simulink model "comparisonModel"  (R2017b)
settings: Solver=VariableStepAuto  StartTime=0.0  StopTime=100  RelTol=1e-3
undefined symbols (not defined in the file): DiscIntNeverNeededParam, sigbuilder_block
settings Model: Creator=Matthias  LastModifiedBy=Kris
settings DebuggingCC: ModelReferenceExtraNoncontSigs=none

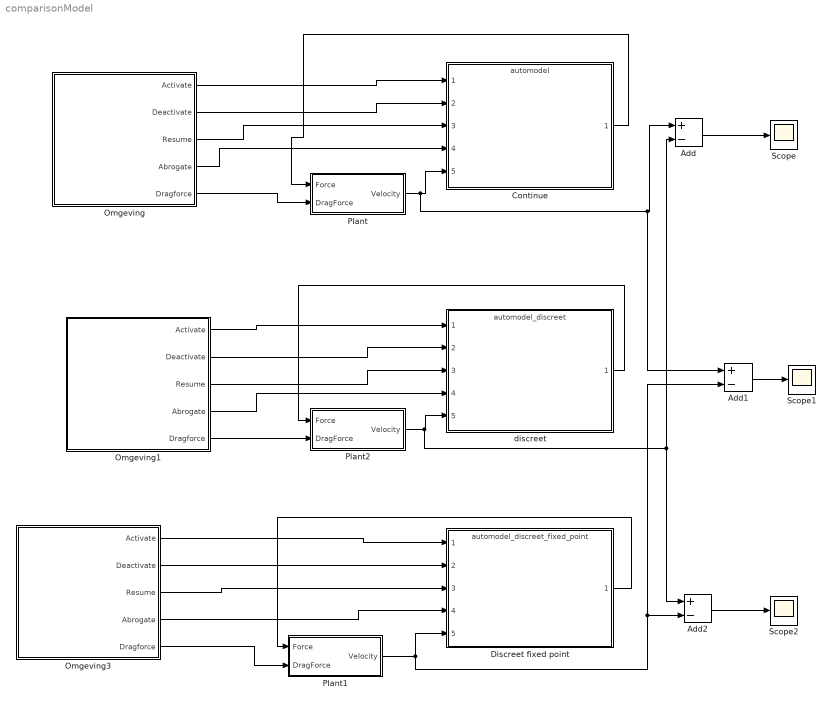
== system comparisonModel ==
  Add : Sum  Inputs=+-
  Add1 : Sum  Inputs=+-
  Add2 : Sum  Inputs=+-
  Continue : ModelReference  ModelNameDialog=automodel.slx  SimulationMode=Normal  ModelReferenceVersion=1.46
  Discreet fixed point : ModelReference  ModelNameDialog=automodel_discreet_fixed_point.slx  SimulationMode=Normal  ModelReferenceVersion=1.55
  Omgeving : Subsystem
  Omgeving1 : Subsystem
  Omgeving3 : Subsystem
  Plant : Subsystem
  Plant1 : Subsystem
  Plant2 : Subsystem
  Scope : Scope
  Scope1 : Scope
  Scope2 : Scope
  discreet : ModelReference  ModelNameDialog=automodel_discreet.slx  SimulationMode=Normal  ModelReferenceVersion=1.47
  wires:
  Omgeving/4(Abrogate) -> Continue/4
  Omgeving/3(Resume) -> Continue/3
  Omgeving/2(Deactivate) -> Continue/2
  Omgeving/1(Activate) -> Continue/1
  Add/1 -> Scope/1
  Add1/1 -> Scope1/1
  Add2/1 -> Scope2/1
  Plant/1(Velocity) -> Add1/1, Add/1, Continue/5
  Plant2/1(Velocity) -> Add/2, Add2/1, discreet/5
  Omgeving1/1(Activate) -> discreet/1
  Omgeving1/2(Deactivate) -> discreet/2
  Omgeving1/3(Resume) -> discreet/3
  Omgeving1/4(Abrogate) -> discreet/4
  Omgeving1/5(Dragforce) -> Plant2/2(DragForce)
  Omgeving/5(Dragforce) -> Plant/2(DragForce)
  Omgeving3/5(Dragforce) -> Plant1/2(DragForce)
  Omgeving3/1(Activate) -> Discreet fixed point/1
  Discreet fixed point/1 -> Plant1/1("Force ")
  Omgeving3/2(Deactivate) -> Discreet fixed point/2
  Omgeving3/4(Abrogate) -> Discreet fixed point/4
  Omgeving3/3(Resume) -> Discreet fixed point/3
  Plant1/1(Velocity) -> Add2/2, Add1/2, Discreet fixed point/5
  discreet/1 -> Plant2/1("Force ")
  Continue/1 -> Plant/1("Force ")

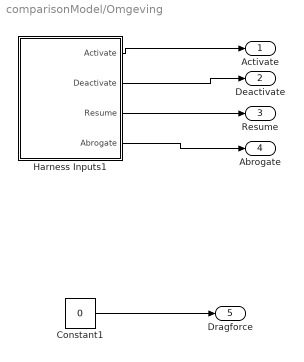
== system comparisonModel/Omgeving ==
  Constant1 : Constant  Value=0
  Harness Inputs1 : Subsystem  Tag=STV Subsys  LoadFcn=sigbuilder_block('load');  StartFcn=sigbuilder_block('start');  StopFcn=sigbuilder_block('stop');  ClipboardFcn=sigbuilder_block('clipboard');  mask(Sigbuilder block){tuvar=[0:10]}
      mask init:
      | if ~strcmp(get_param(bdroot(gcb),'SimulationStatus'),'stopped'),tuvar = sigbuilder_block('maskInit'); end
      settings: CopyFcn=sigbuilder_block('copy');  DeleteFcn=sigbuilder_block('delete');  ModelCloseFcn=sigbuilder_block('modelClose');  PreSaveFcn=sigbuilder_block('preSave');  PauseFcn=sigbuilder_block('pause');  ContinueFcn=sigbuilder_block('continue');  NameChangeFcn=sigbuilder_block('namechange');  OpenFcn=sigbuilder_block('open',[50.25 50.25 878.25 399.75 ]);  CloseFcn=sigbuilder_block('close');
      mask Display: plot(0, 0, 100, 100,[2, 2, 32, 32, 2], [68, 8, 8, 68, 68],[32, 2], [38, 38], [32, 19, 2],[53, 60, 44], [32, 17, 17, 2],[16, 16, 31, 31]);txt = getActiveGroup(gcbh);text(2, 100, txt,'verticalAlignment', 'top');
  Activate : Outport
  Deactivate : Outport  Port=2
  Resume : Outport  Port=3
  Abrogate : Outport  Port=4
  Dragforce : Outport  Port=5
  wires:
  Harness Inputs1/1(Activate) -> Activate/1
  Harness Inputs1/2(Deactivate) -> Deactivate/1
  Harness Inputs1/3(Resume) -> Resume/1
  Harness Inputs1/4(Abrogate) -> Abrogate/1
  Constant1/1 -> Dragforce/1

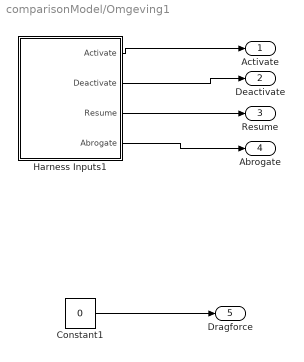
== system comparisonModel/Omgeving1 ==
  Constant1 : Constant  Value=0
  Harness Inputs1 : Subsystem  Tag=STV Subsys  LoadFcn=sigbuilder_block('load');  StartFcn=sigbuilder_block('start');  StopFcn=sigbuilder_block('stop');  ClipboardFcn=sigbuilder_block('clipboard');  mask(Sigbuilder block){tuvar=[0:10]}
      mask init:
      | if ~strcmp(get_param(bdroot(gcb),'SimulationStatus'),'stopped'),tuvar = sigbuilder_block('maskInit'); end
      settings: CopyFcn=sigbuilder_block('copy');  DeleteFcn=sigbuilder_block('delete');  ModelCloseFcn=sigbuilder_block('modelClose');  PreSaveFcn=sigbuilder_block('preSave');  PauseFcn=sigbuilder_block('pause');  ContinueFcn=sigbuilder_block('continue');  NameChangeFcn=sigbuilder_block('namechange');  OpenFcn=sigbuilder_block('open',[50.25 50.25 878.25 399.75 ]);  CloseFcn=sigbuilder_block('close');
      mask Display: plot(0, 0, 100, 100,[2, 2, 32, 32, 2], [68, 8, 8, 68, 68],[32, 2], [38, 38], [32, 19, 2],[53, 60, 44], [32, 17, 17, 2],[16, 16, 31, 31]);txt = getActiveGroup(gcbh);text(2, 100, txt,'verticalAlignment', 'top');
  Activate : Outport
  Deactivate : Outport  Port=2
  Resume : Outport  Port=3
  Abrogate : Outport  Port=4
  Dragforce : Outport  Port=5
  wires:
  Harness Inputs1/1(Activate) -> Activate/1
  Harness Inputs1/2(Deactivate) -> Deactivate/1
  Harness Inputs1/3(Resume) -> Resume/1
  Harness Inputs1/4(Abrogate) -> Abrogate/1
  Constant1/1 -> Dragforce/1

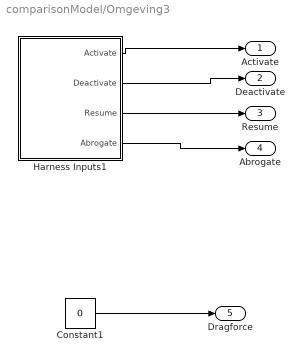
== system comparisonModel/Omgeving3 ==
  Constant1 : Constant  Value=0
  Harness Inputs1 : Subsystem  Tag=STV Subsys  LoadFcn=sigbuilder_block('load');  StartFcn=sigbuilder_block('start');  StopFcn=sigbuilder_block('stop');  ClipboardFcn=sigbuilder_block('clipboard');  mask(Sigbuilder block){tuvar=[0:10]}
      mask init:
      | if ~strcmp(get_param(bdroot(gcb),'SimulationStatus'),'stopped'),tuvar = sigbuilder_block('maskInit'); end
      settings: CopyFcn=sigbuilder_block('copy');  DeleteFcn=sigbuilder_block('delete');  ModelCloseFcn=sigbuilder_block('modelClose');  PreSaveFcn=sigbuilder_block('preSave');  PauseFcn=sigbuilder_block('pause');  ContinueFcn=sigbuilder_block('continue');  NameChangeFcn=sigbuilder_block('namechange');  OpenFcn=sigbuilder_block('open',[50.25 50.25 878.25 399.75 ]);  CloseFcn=sigbuilder_block('close');
      mask Display: plot(0, 0, 100, 100,[2, 2, 32, 32, 2], [68, 8, 8, 68, 68],[32, 2], [38, 38], [32, 19, 2],[53, 60, 44], [32, 17, 17, 2],[16, 16, 31, 31]);txt = getActiveGroup(gcbh);text(2, 100, txt,'verticalAlignment', 'top');
  Activate : Outport
  Deactivate : Outport  Port=2
  Resume : Outport  Port=3
  Abrogate : Outport  Port=4
  Dragforce : Outport  Port=5
  wires:
  Harness Inputs1/1(Activate) -> Activate/1
  Harness Inputs1/2(Deactivate) -> Deactivate/1
  Harness Inputs1/3(Resume) -> Resume/1
  Harness Inputs1/4(Abrogate) -> Abrogate/1
  Constant1/1 -> Dragforce/1

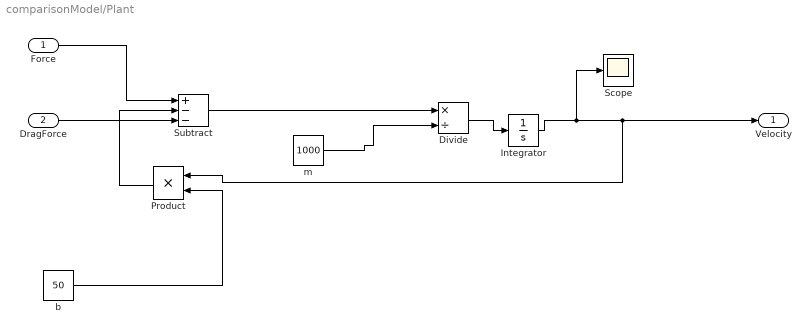
== system comparisonModel/Plant ==
  "Force " : Inport
  DragForce : Inport  Port=2
  Divide : Product  Inputs=*/
  Integrator : Integrator
  Product : Product
  Scope : Scope
  Subtract : Sum  Inputs=+--
  b : Constant  Value=50
  m : Constant  Value=1000
  Velocity : Outport
  wires:
  Product/1 -> Subtract/2
  b/1 -> Product/2
  Subtract/1 -> Divide/1
  "Force "/1 -> Subtract/1
  Divide/1 -> Integrator/1
  m/1 -> Divide/2
  DragForce/1 -> Subtract/3
  Integrator/1 -> Scope/1, Product/1, Velocity/1

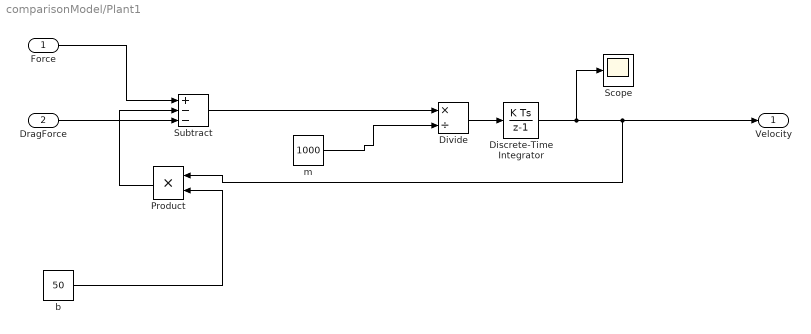
== system comparisonModel/Plant1 ==
  "Force " : Inport
  DragForce : Inport  Port=2
  Discrete-Time Integrator : DiscreteIntegrator  InitialConditionSetting=State (most efficient)  SampleTime=-1  OutDataTypeStr=Inherit: Inherit via back propagation  ICPrevOutput=DiscIntNeverNeededParam  ICPrevScaledInput=DiscIntNeverNeededParam
  Divide : Product  Inputs=*/  OutDataTypeStr=Inherit: Inherit via back propagation
  Product : Product
  Scope : Scope
  Subtract : Sum  Inputs=+--
  b : Constant  Value=50  OutDataTypeStr=fixdt(1,32,0)
  m : Constant  Value=1000
  Velocity : Outport
  wires:
  Product/1 -> Subtract/2
  b/1 -> Product/2
  Subtract/1 -> Divide/1
  "Force "/1 -> Subtract/1
  Divide/1 -> Discrete-Time Integrator/1
  m/1 -> Divide/2
  DragForce/1 -> Subtract/3
  Discrete-Time Integrator/1 -> Scope/1, Product/1, Velocity/1

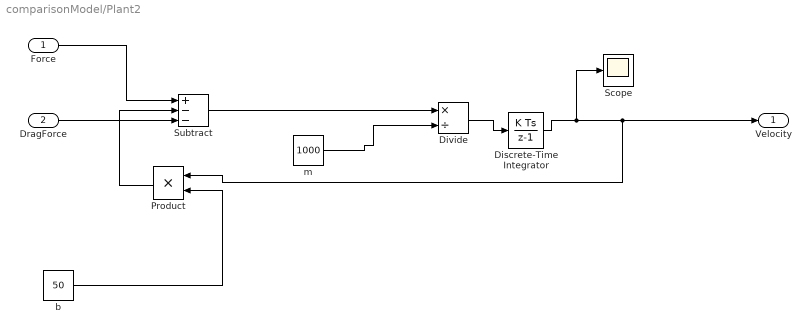
== system comparisonModel/Plant2 ==
  "Force " : Inport
  DragForce : Inport  Port=2
  Discrete-Time Integrator : DiscreteIntegrator  InitialConditionSetting=State (most efficient)  SampleTime=-1  ICPrevOutput=DiscIntNeverNeededParam  ICPrevScaledInput=DiscIntNeverNeededParam
  Divide : Product  Inputs=*/
  Product : Product
  Scope : Scope
  Subtract : Sum  Inputs=+--
  b : Constant  Value=50
  m : Constant  Value=1000
  Velocity : Outport
  wires:
  Product/1 -> Subtract/2
  b/1 -> Product/2
  Subtract/1 -> Divide/1
  "Force "/1 -> Subtract/1
  Divide/1 -> Discrete-Time Integrator/1
  m/1 -> Divide/2
  DragForce/1 -> Subtract/3
  Discrete-Time Integrator/1 -> Scope/1, Product/1, Velocity/1

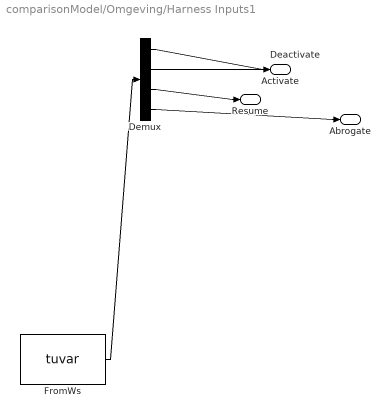
== system comparisonModel/Omgeving/Harness Inputs1 ==
  Demux : Demux  Tag=STV Demux
  FromWs : FromWorkspace  Tag=STV FromWs  VariableName=tuvar  SampleTime=0
      SigBuilderData=|
      | dataSet.timeRange = [0 200]
      | dataSet.name = 'Group 1'
      | sbobj.Name = 'Signal Builder'
      | sbobj.Groups.Name = 'Group 1'
      | sbobj.Groups.Signals(1).Name = 'Activate'
      | sbobj.Groups.Signals(1).XData = [0 7.2 7.2 200]
      | sbobj.Groups.Signals(1).YData = [0 0 1 1]
      | sbobj.Groups.Signals(2).Name = 'Deactivate'
      | sbobj.Groups.Signals(2).XData = [0 0.1 200]
      | sbobj.Groups.Signals(2).YData = [0 0 0]
      | sbobj.Groups.Signals(3).Name = 'Resume'
      | sbobj.Groups.Signals(3).XData = [0 200]
      | sbobj.Groups.Signals(3).YData = [0 0]
      | sbobj.Groups.Signals(4).Name = 'Abrogate'
      | sbobj.Groups.Signals(4).XData = [0 200]
      | sbobj.Groups.Signals(4).YData = [0 0]
      | sbobj.Groups.TimeRange = [0 200]
  Activate : Outport  Tag=STV Outport
  Deactivate : Outport  Tag=STV Outport  Port=2
  Resume : Outport  Tag=STV Outport  Port=3
  Abrogate : Outport  Tag=STV Outport  Port=4
  wires:
  FromWs/1 -> Demux/1
  Demux/1 -> Activate/1
  Demux/2 -> Deactivate/1
  Demux/3 -> Resume/1
  Demux/4 -> Abrogate/1

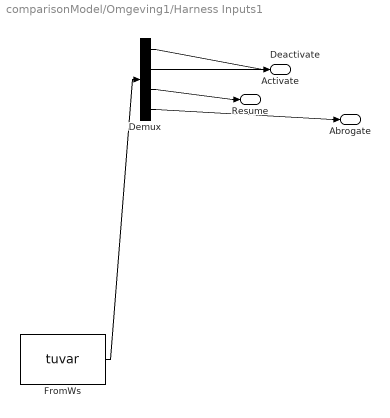
== system comparisonModel/Omgeving1/Harness Inputs1 ==
  Demux : Demux  Tag=STV Demux
  FromWs : FromWorkspace  Tag=STV FromWs  VariableName=tuvar  SampleTime=0
      SigBuilderData=|
      | dataSet.timeRange = [0 200]
      | dataSet.name = 'Group 1'
      | sbobj.Name = 'Signal Builder'
      | sbobj.Groups.Name = 'Group 1'
      | sbobj.Groups.Signals(1).Name = 'Activate'
      | sbobj.Groups.Signals(1).XData = [0 7.2 7.2 200]
      | sbobj.Groups.Signals(1).YData = [0 0 1 1]
      | sbobj.Groups.Signals(2).Name = 'Deactivate'
      | sbobj.Groups.Signals(2).XData = [0 0.1 200]
      | sbobj.Groups.Signals(2).YData = [0 0 0]
      | sbobj.Groups.Signals(3).Name = 'Resume'
      | sbobj.Groups.Signals(3).XData = [0 200]
      | sbobj.Groups.Signals(3).YData = [0 0]
      | sbobj.Groups.Signals(4).Name = 'Abrogate'
      | sbobj.Groups.Signals(4).XData = [0 200]
      | sbobj.Groups.Signals(4).YData = [0 0]
      | sbobj.Groups.TimeRange = [0 200]
  Activate : Outport  Tag=STV Outport
  Deactivate : Outport  Tag=STV Outport  Port=2
  Resume : Outport  Tag=STV Outport  Port=3
  Abrogate : Outport  Tag=STV Outport  Port=4
  wires:
  FromWs/1 -> Demux/1
  Demux/1 -> Activate/1
  Demux/2 -> Deactivate/1
  Demux/3 -> Resume/1
  Demux/4 -> Abrogate/1

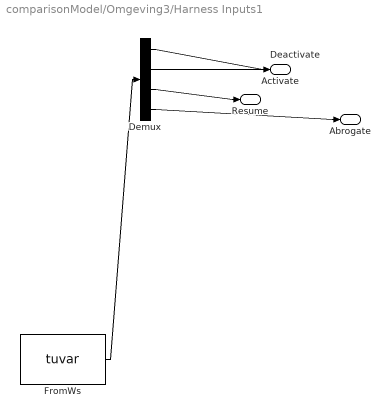
== system comparisonModel/Omgeving3/Harness Inputs1 ==
  Demux : Demux  Tag=STV Demux
  FromWs : FromWorkspace  Tag=STV FromWs  VariableName=tuvar  SampleTime=0
      SigBuilderData=|
      | dataSet.timeRange = [0 200]
      | dataSet.name = 'Group 1'
      | sbobj.Name = 'Signal Builder'
      | sbobj.Groups.Name = 'Group 1'
      | sbobj.Groups.Signals(1).Name = 'Activate'
      | sbobj.Groups.Signals(1).XData = [0 7.2 7.2 200]
      | sbobj.Groups.Signals(1).YData = [0 0 1 1]
      | sbobj.Groups.Signals(2).Name = 'Deactivate'
      | sbobj.Groups.Signals(2).XData = [0 0.1 200]
      | sbobj.Groups.Signals(2).YData = [0 0 0]
      | sbobj.Groups.Signals(3).Name = 'Resume'
      | sbobj.Groups.Signals(3).XData = [0 200]
      | sbobj.Groups.Signals(3).YData = [0 0]
      | sbobj.Groups.Signals(4).Name = 'Abrogate'
      | sbobj.Groups.Signals(4).XData = [0 200]
      | sbobj.Groups.Signals(4).YData = [0 0]
      | sbobj.Groups.TimeRange = [0 200]
  Activate : Outport  Tag=STV Outport
  Deactivate : Outport  Tag=STV Outport  Port=2
  Resume : Outport  Tag=STV Outport  Port=3
  Abrogate : Outport  Tag=STV Outport  Port=4
  wires:
  FromWs/1 -> Demux/1
  Demux/1 -> Activate/1
  Demux/2 -> Deactivate/1
  Demux/3 -> Resume/1
  Demux/4 -> Abrogate/1
